simulink model "HuiL_HVAC_all"  (R2017a)
settings: Solver=VariableStepAuto  StartTime=0.0  StopTime=1000  RelTol=1e-3
values from neighbouring files (symbols this model uses):
  A_bdy = 0.202 * body_weight^0.425 * body_height^0.725    (= 2.36373135571)    [HuiL_HVAC_mdl_all_sim.m]
  activities = struct(args{:})    [HuiL_HVAC_mdl_all_sim.m]
  activity_0 = 'sit'    [HuiL_HVAC_mdl_all_sim.m]
  activity_1 = 'sit'    [HuiL_HVAC_mdl_all_sim.m]
  activity_t = activity_t_tmp    (= 0)    [HuiL_HVAC_mdl_all_sim.m]
  clothing_0 = 'office_t'    [HuiL_HVAC_mdl_all_sim.m]
  clothing_1 = 'office_t'    [HuiL_HVAC_mdl_all_sim.m]
  clothing_t = clothing_t_tmp    (= 0)    [HuiL_HVAC_mdl_all_sim.m]
  clothings = struct(args{:})    [HuiL_HVAC_mdl_all_sim.m]
  cp_body = 4180    [HuiL_HVAC_mdl_all_sim.m]
  eta_4_thresh = 50    [HuiL_HVAC_mdl_all_sim.m]
  in_out_0 = 1    [HuiL_HVAC_mdl_all_sim.m]
  in_out_1 = 2    [HuiL_HVAC_mdl_all_sim.m]
  in_out_t = in_out_t_tmp    (= 0)    [HuiL_HVAC_mdl_all_sim.m]
  k_comf = 50    [HuiL_HVAC_mdl_all_sim.m]
  k_dT = 1.    (= 1)    [HuiL_HVAC_mdl_all_sim.m]
  m_body = 100    [HuiL_HVAC_mdl_all_sim.m]
  T_b_0 = tmp_T_b(end,:)    [HuiL_HVAC_mdl_all_sim.m]
  T_b_ref = 37    [HuiL_HVAC_mdl_all_sim.m]
  T_out = 10    [HuiL_HVAC_mdl_all_sim.m]
  T_r_db = 1    [HuiL_HVAC_mdl_all_sim.m]
  T_r_ref_0 = tmp_T_r_ref(end,:)'    [HuiL_HVAC_mdl_all_sim.m]
  t_xi_2_off = t_xi_2_off_tmp    (= 14)    [HuiL_HVAC_mdl_all_sim.m]
  t_xi_2_on = t_xi_2_on_tmp    (= 7)    [HuiL_HVAC_mdl_all_sim.m]
  t_xi_3_off = t_xi_3_off_tmp    (= 14)    [HuiL_HVAC_mdl_all_sim.m]
  t_xi_3_on = t_xi_3_on_tmp    (= 7)    [HuiL_HVAC_mdl_all_sim.m]
  t_xi_5_off = t_xi_5_off_tmp    (= 14)    [HuiL_HVAC_mdl_all_sim.m]
  t_xi_5_on = t_xi_5_on_tmp    (= 7)    [HuiL_HVAC_mdl_all_sim.m]
  t_xi_8_off = t_xi_8_off_tmp    (= 0)    [HuiL_HVAC_mdl_all_sim.m]
  t_xi_8_on = t_xi_8_on_tmp    (= 0)    [HuiL_HVAC_mdl_all_sim.m]
  xi_1_0 = 3    [HuiL_HVAC_mdl_all_sim.m]
  xi_2_0 = 5    [HuiL_HVAC_mdl_all_sim.m]
  xi_2_on = 5    [HuiL_HVAC_mdl_all_sim.m]
  xi_3_0 = 5    [HuiL_HVAC_mdl_all_sim.m]
  xi_3_on = 5    [HuiL_HVAC_mdl_all_sim.m]
  xi_4_0 = 0    [HuiL_HVAC_mdl_all_sim.m]
  xi_5_0 = 3    [HuiL_HVAC_mdl_all_sim.m]
  xi_5_on = 3    [HuiL_HVAC_mdl_all_sim.m]
  xi_6_phi = 0.6    [HuiL_HVAC_mdl_all_sim.m]
  xi_6_var = 0    [HuiL_HVAC_mdl_all_sim.m]
  xi_7_phi = 0.8    [HuiL_HVAC_mdl_all_sim.m]
  xi_7_var = 0    [HuiL_HVAC_mdl_all_sim.m]
  xi_8_0 = 0    [HuiL_HVAC_mdl_all_sim.m]
  xi_8_on = 0    [HuiL_HVAC_mdl_all_sim.m]
libraries: dspsigops x1
settings Model: Creator=thisi  LastModifiedBy=thisi
settings DataIOCC: ReturnWorkspaceOutputs=on

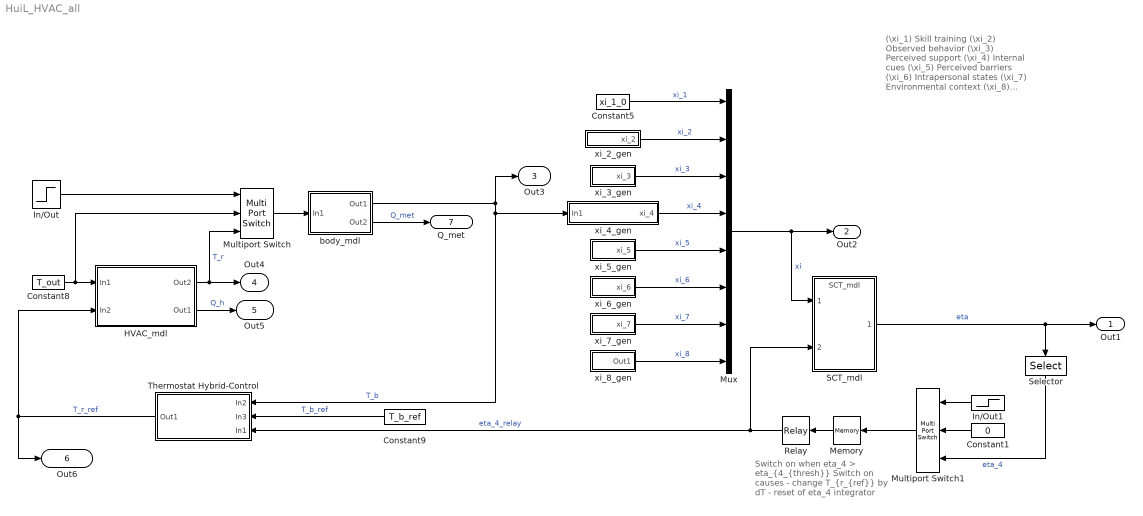
== system HuiL_HVAC_all ==
  note: (\xi_1) Skill training
      | (\xi_2) Observed behavior
      | (\xi_3) Perceived support
      | (\xi_4) Internal cues
      | (\xi_5) Perceived barriers
      | (\xi_6) Intrapersonal states
      | (\xi_7) Environmental context
      | (\xi_8) External cues
      |
      | (\eta_1) Self-management skills
      | (\eta_2) Outcome expectancy
      | (\eta_3) Self-efficacy
      | (\eta_4) Behavior
      | (\eta_5) Behavioral outcomes
      | (\eta_6) Cue to action
      |
      | (T_b) Body temperature
      | (T_{b_{ref}}) Body temperature setpoint
      |
      | (T_r) Room temperature
      | (T_{r_{ref}}) Room thermostat setpoint
  note: Switch on when eta_4 > eta_{4_{thresh}}
      | Switch on causes
      |  - change T_{r_{ref}} by dT
      |  - reset of eta_4 integrator
  Constant1 : Constant  Value=0
  Constant5 : Constant  Value=xi_1_0
  Constant8 : Constant  Value=T_out
  Constant9 : Constant  Value=T_b_ref
  HVAC_mdl : Subsystem
  In/Out : Step  Time=in_out_t  Before=in_out_0  After=in_out_1  SampleTime=0
  In/Out1 : Step  Time=in_out_t  Before=in_out_0  After=in_out_1  SampleTime=0
  Memory : Memory
  Multiport Switch : MultiPortSwitch  Inputs=2
  Multiport Switch1 : MultiPortSwitch  Inputs=2
  Mux : Mux  Inputs=8
  Relay : Relay  OnSwitchValue=min(eta_4_thresh * 1.01, 100-eps)  OffSwitchValue=eta_4_thresh * 0.99
  SCT_mdl : ModelReference  ModelNameDialog=SCT_mdl.slx  SimulationMode=Normal  ModelReferenceVersion=1.3
  Selector : Selector  InputPortWidth=6  IndexOptions=Index vector (dialog)  Indices=4  OutputSizes=1
  Thermostat Hybrid-Control : Subsystem  VariantControl=VSS_thermostat==1
  body_mdl : Subsystem
  xi_2_gen : Subsystem  VariantControl=VSS_xi_8_gen_switch
  xi_3_gen : Subsystem
  xi_4_gen : Subsystem  Variant=on
  xi_5_gen : Subsystem
  xi_6_gen : Subsystem
  xi_7_gen : Subsystem
  xi_8_gen : Subsystem
  Out1 : Outport
  Out2 : Outport  Port=2
  Out3 : Outport  Port=3
  Out4 : Outport  Port=4
  Out5 : Outport  Port=5
  Out6 : Outport  Port=6
  Q_met : Outport  Port=7
  wires:
  Mux/1 -> SCT_mdl/1, Out2/1  "xi"
  SCT_mdl/1 -> Selector/1, Out1/1  "eta"
  xi_5_gen/1(xi_5) -> Mux/5  "xi_5"
  xi_4_gen/1(xi_4) -> Mux/4  "xi_4"
  xi_3_gen/1(xi_3) -> Mux/3  "xi_3"
  xi_2_gen/1(xi_2) -> Mux/2  "xi_2"
  Constant5/1 -> Mux/1  "xi_1"
  HVAC_mdl/1(Out2) -> Out4/1, Multiport Switch/3  "T_r"
  body_mdl/1(Out1) -> Thermostat Hybrid-Control/1(In2), xi_4_gen/1(In1), Out3/1  "T_b"
  Constant9/1 -> Thermostat Hybrid-Control/2(In3)  "T_b_ref"
  xi_8_gen/1(Out1) -> Mux/8  "xi_8"
  Constant8/1 -> Multiport Switch/2, HVAC_mdl/1(In1)
  Thermostat Hybrid-Control/1(Out1) -> HVAC_mdl/2(In2), Out6/1  "T_r_ref"
  HVAC_mdl/2(Out1) -> Out5/1  "Q_h"
  xi_6_gen/1(xi_6) -> Mux/6  "xi_6"
  xi_7_gen/1(xi_7) -> Mux/7  "xi_7"
  Memory/1 -> Relay/1
  Selector/1 -> Multiport Switch1/3  "eta_4"
  Multiport Switch/1 -> body_mdl/1(In1)
  In/Out/1 -> Multiport Switch/1
  Relay/1 -> Thermostat Hybrid-Control/3(In1), SCT_mdl/2  "eta_4_relay"
  In/Out1/1 -> Multiport Switch1/1
  Constant1/1 -> Multiport Switch1/2
  Multiport Switch1/1 -> Memory/1
  body_mdl/2(Out2) -> Q_met/1  "Q_met"

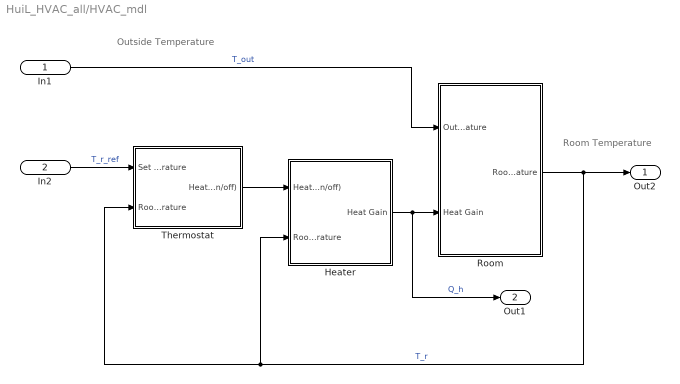
== system HuiL_HVAC_all/HVAC_mdl ==
  note: Outside
      | Temperature
  note: Room
      | Temperature
  In1 : Inport  Unit=°C
  In2 : Inport  Port=2  Unit=°C
  Heater : Subsystem
  Room : Subsystem
  Thermostat : Subsystem
  Out2 : Outport  Unit=°C
  Out1 : Outport  Port=2  Unit=joule/hour
  wires:
  In1/1 -> Room/1(Outside Temperature)  "T_out"
  Heater/1(Heat Gain) -> Out1/1, Room/2("Heat Gain ")  "Q_h"
  Thermostat/1(Heater (on/off)) -> Heater/1(Heater (on/off))
  Room/1(Room Temperature) -> Out2/1, Heater/2(Room Temperature), Thermostat/2("    Room Temperature")  "T_r"
  In2/1 -> Thermostat/1(Set Room Temperature)  "T_r_ref"

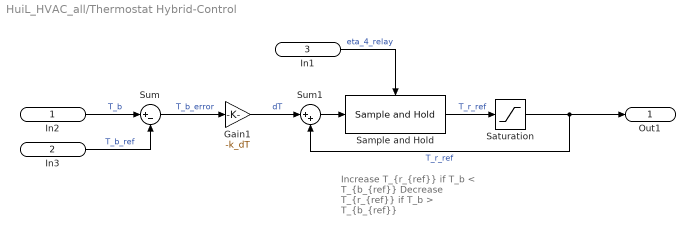
== system HuiL_HVAC_all/Thermostat Hybrid-Control ==
  note: Increase T_{r_{ref}} if T_b < T_{b_{ref}}
      | Decrease T_{r_{ref}} if T_b > T_{b_{ref}}
  In2 : Inport
  In3 : Inport  Port=2
  In1 : Inport  Port=3
  Gain1 : Gain  Gain=-k_dT
      settings: AttributesFormatString=%<Gain>
  Sample and Hold : dspsigops/Sample and Hold  trig=Rising edge  initCond=T_r_ref_0  latchinput=on
  Saturation : Saturate  UpperLimit=35  LowerLimit=10
  Sum : Sum  Inputs=|+-
  Sum1 : Sum  Inputs=|++
  Out1 : Outport  InitialOutput=T_r_ref_0
  wires:
  In3/1 -> Sum/2  "T_b_ref"
  In2/1 -> Sum/1  "T_b"
  Sum/1 -> Gain1/1  "T_b_error"
  Sample and Hold/1 -> Saturation/1  "T_r_ref"
  In1/1 -> Sample and Hold/Trigger  "eta_4_relay"
  Sum1/1 -> Sample and Hold/1
  Gain1/1 -> Sum1/1  "dT"
  Saturation/1 -> Out1/1, Sum1/2  "T_r_ref"

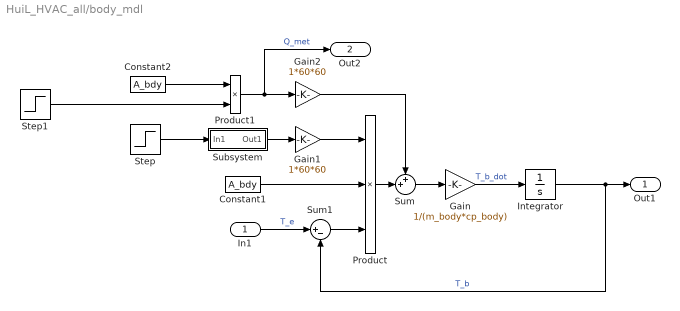
== system HuiL_HVAC_all/body_mdl ==
  In1 : Inport
  Constant1 : Constant  Value=A_bdy
  Constant2 : Constant  Value=A_bdy
  Gain : Gain  Gain=1/(m_body*cp_body)
      settings: AttributesFormatString=%<Gain>
  Gain1 : Gain  Gain=1*60*60
      settings: AttributesFormatString=W to J/hr
  Gain2 : Gain  Gain=1*60*60
      settings: AttributesFormatString=W to J/hr
  Integrator : Integrator  InitialCondition=T_b_0
  Product : Product  Inputs=3
  Product1 : Product
  Step : Step  Time=clothing_t  Before=clothings.(clothing_0).val  After=clothings.(clothing_1).val  SampleTime=0
      settings: AttributesFormatString=|
      | %<Time>
      | %<Before>
      | %<After>
  Step1 : Step  Time=activity_t  Before=activities.(activity_0).val  After=activities.(activity_1).val  SampleTime=0
      settings: AttributesFormatString=|
      | %<Time>
      | %<Before>
      | %<After>
  Subsystem : Subsystem
  Sum : Sum  Inputs=++|
  Sum1 : Sum  Inputs=|+-
  Out1 : Outport
  Out2 : Outport  Port=2
  wires:
  Sum1/1 -> Product/3
  Gain/1 -> Integrator/1  "T_b_dot"
  Integrator/1 -> Out1/1, Sum1/2  "T_b"
  Sum/1 -> Gain/1
  Constant1/1 -> Product/2
  In1/1 -> Sum1/1  "T_e"
  Step/1 -> Subsystem/1(In1)
  Product/1 -> Sum/2
  Step1/1 -> Product1/2
  Gain1/1 -> Product/1
  Gain2/1 -> Sum/1
  Subsystem/1(Out1) -> Gain1/1
  Constant2/1 -> Product1/1
  Product1/1 -> Out2/1, Gain2/1  "Q_met"

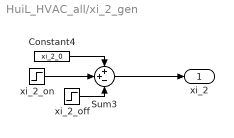
== system HuiL_HVAC_all/xi_2_gen ==
  Constant4 : Constant  Value=xi_2_0
  Sum3 : Sum  Inputs=++-
  xi_2_off : Step  Time=t_xi_2_off  After=xi_2_on - xi_2_0  SampleTime=0
  xi_2_on : Step  Time=t_xi_2_on  After=xi_2_on - xi_2_0  SampleTime=0
  xi_2 : Outport
  wires:
  Constant4/1 -> Sum3/1
  Sum3/1 -> xi_2/1
  xi_2_on/1 -> Sum3/2
  xi_2_off/1 -> Sum3/3

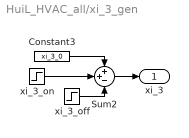
== system HuiL_HVAC_all/xi_3_gen ==
  Constant3 : Constant  Value=xi_3_0
  Sum2 : Sum  Inputs=++-
  xi_3_off : Step  Time=t_xi_3_off  After=xi_3_on - xi_3_0  SampleTime=0
  xi_3_on : Step  Time=t_xi_3_on  After=xi_3_on - xi_3_0  SampleTime=0
  xi_3 : Outport
  wires:
  xi_3_on/1 -> Sum2/2
  xi_3_off/1 -> Sum2/3
  Constant3/1 -> Sum2/1
  Sum2/1 -> xi_3/1

== system HuiL_HVAC_all/xi_4_gen ==
  note: 1) Add Subsystem or Model blocks as valid variant choices.
      | 2) You cannot connect blocks at this level. At simulation, connectivity is automatically
      | determined, based on the active variant and port name matching.
  In1 : Inport
  Body : Subsystem  VariantControl=VSS_xi_4_gen==2
  Const : Subsystem  VariantControl=VSS_xi_4_gen==1
  xi_4 : Outport

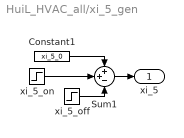
== system HuiL_HVAC_all/xi_5_gen ==
  Constant1 : Constant  Value=xi_5_0
  Sum1 : Sum  Inputs=++-
  xi_5_off : Step  Time=t_xi_5_off  After=xi_5_on - xi_5_0  SampleTime=0
  xi_5_on : Step  Time=t_xi_5_on  After=xi_5_on - xi_5_0  SampleTime=0
  xi_5 : Outport
  wires:
  Constant1/1 -> Sum1/1
  xi_5_off/1 -> Sum1/3
  xi_5_on/1 -> Sum1/2
  Sum1/1 -> xi_5/1

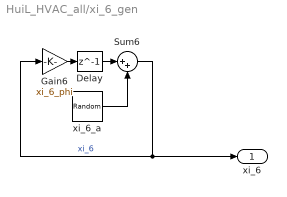
== system HuiL_HVAC_all/xi_6_gen ==
  Delay : Delay  DelayLength=1
  Gain6 : Gain  Gain=xi_6_phi
      settings: AttributesFormatString=%<Gain>
  Sum6 : Sum  Inputs=|++
  xi_6_a : RandomNumber  Variance=xi_6_var  SampleTime=0.1
  xi_6 : Outport
  wires:
  Delay/1 -> Sum6/1
  Sum6/1 -> xi_6/1, Gain6/1  "xi_6"
  xi_6_a/1 -> Sum6/2
  Gain6/1 -> Delay/1

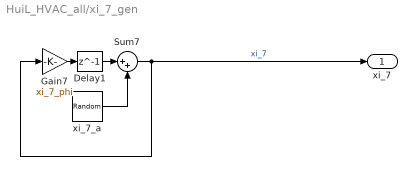
== system HuiL_HVAC_all/xi_7_gen ==
  Delay1 : Delay  DelayLength=1
  Gain7 : Gain  Gain=xi_7_phi
      settings: AttributesFormatString=%<Gain>
  Sum7 : Sum  Inputs=|++
  xi_7_a : RandomNumber  Variance=xi_7_var  SampleTime=0.1
  xi_7 : Outport
  wires:
  Gain7/1 -> Delay1/1
  xi_7_a/1 -> Sum7/2
  Delay1/1 -> Sum7/1
  Sum7/1 -> xi_7/1, Gain7/1  "xi_7"

== system HuiL_HVAC_all/xi_8_gen ==
  Constant : Constant  Value=xi_8_0
  Sum : Sum  Inputs=++-
  xi_8_off : Step  Time=t_xi_8_off  After=xi_8_on - xi_8_0  SampleTime=0
  xi_8_on : Step  Time=t_xi_8_on  After=xi_8_on - xi_8_0  SampleTime=0
  Out1 : Outport
  wires:
  xi_8_off/1 -> Sum/3
  xi_8_on/1 -> Sum/2
  Constant/1 -> Sum/1
  Sum/1 -> Out1/1  "xi_8"

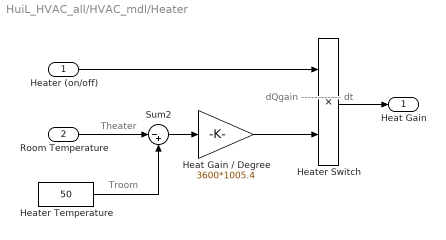
== system HuiL_HVAC_all/HVAC_mdl/Heater ==
  note: dQgain
      | ------------
      |    dt
  note: Troom
  note: Theater
  Heater (on/off) : Inport
  Room Temperature : Inport  Port=2
  Heat Gain / Degree : Gain  Gain=3600*1005.4
  Heater Switch : Product  RndMeth=Zero
  Heater Temperature : Constant  Value=50
  Sum2 : Sum  Inputs=|-+
  Heat Gain : Outport  Unit=joule/hour
  wires:
  Heater Temperature/1 -> Sum2/2
  Room Temperature/1 -> Sum2/1
  Sum2/1 -> Heat Gain / Degree/1
  Heat Gain / Degree/1 -> Heater Switch/2
  Heater (on/off)/1 -> Heater Switch/1
  Heater Switch/1 -> Heat Gain/1

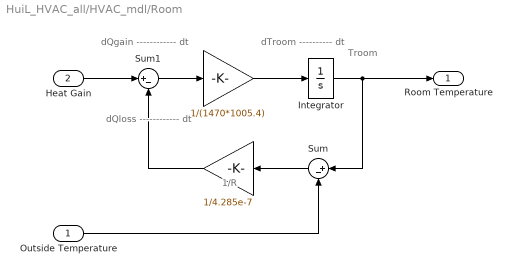
== system HuiL_HVAC_all/HVAC_mdl/Room ==
  note: 1/R
  note: Troom
  note: dQloss
      | ------------
      |      dt
  note: dQgain
      | ------------
      |      dt
  note: dTroom
      | ----------
      |     dt
  Outside Temperature : Inport  Unit=°C
  "Heat Gain " : Inport  Port=2  Unit=joule/h
  " " : Gain  Gain=1/4.285e-7  SaturateOnIntegerOverflow=on  OutDataTypeStr=Inherit: Same as input  ParamDataTypeStr=Inherit: Same as input
      settings: AttributesFormatString=%<Gain>
  "  " : Gain  Gain=1/(1470*1005.4)  SaturateOnIntegerOverflow=on  OutDataTypeStr=Inherit: Same as input  ParamDataTypeStr=Inherit: Same as input
      settings: AttributesFormatString=%<Gain>
  Integrator : Integrator  InitialCondition=20
  Sum : Sum  Inputs=|+-
  Sum1 : Sum  Inputs=|+-  SaturateOnIntegerOverflow=on  InputSameDT=on  OutDataTypeStr=Inherit: Same as first input
  Room Temperature : Outport  Unit=°C
  wires:
  "Heat Gain "/1 -> Sum1/1
  Sum1/1 -> "  "/1
  "  "/1 -> Integrator/1
  Integrator/1 -> Sum/1, Room Temperature/1
  " "/1 -> Sum1/2
  Sum/1 -> " "/1
  Outside Temperature/1 -> Sum/2

== system HuiL_HVAC_all/HVAC_mdl/Thermostat ==
  Set Room Temperature : Inport
  "    Room Temperature" : Inport  Port=2
  Relay1 : Relay  OnSwitchValue=T_r_db  OffSwitchValue=-T_r_db
  Sum : Sum  Inputs=|+-  SaturateOnIntegerOverflow=on  InputSameDT=on  OutDataTypeStr=Inherit: Same as first input
  Heater (on/off) : Outport
  wires:
  Set Room Temperature/1 -> Sum/1
  Relay1/1 -> Heater (on/off)/1
  Sum/1 -> Relay1/1
  "    Room Temperature"/1 -> Sum/2

== system HuiL_HVAC_all/body_mdl/Subsystem ==
  In1 : Inport
  Gain3 : Gain  Gain=1/0.155
      settings: AttributesFormatString=%<Gain>
  Math Function : Math  Operator=reciprocal  SaturateOnIntegerOverflow=on
  Out1 : Outport
  wires:
  In1/1 -> Math Function/1  "I_cl"
  Gain3/1 -> Out1/1  "h_bdy"
  Math Function/1 -> Gain3/1

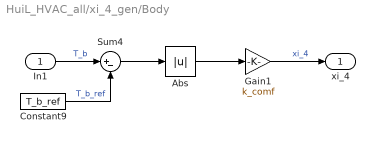
== system HuiL_HVAC_all/xi_4_gen/Body ==
  In1 : Inport
  Abs : Abs
  Constant9 : Constant  Value=T_b_ref
  Gain1 : Gain  Gain=k_comf
      settings: AttributesFormatString=%<Gain>
  Sum4 : Sum  Inputs=|+-
  xi_4 : Outport
  wires:
  Constant9/1 -> Sum4/2  "T_b_ref"
  Sum4/1 -> Abs/1
  Abs/1 -> Gain1/1
  In1/1 -> Sum4/1  "T_b"
  Gain1/1 -> xi_4/1  "xi_4"

== system HuiL_HVAC_all/xi_4_gen/Const ==
  Constant2 : Constant  Value=xi_4_0
  xi_4 : Outport
  wires:
  Constant2/1 -> xi_4/1  "xi_4"
